simulink model "Basic_Control_Pendulum_RBF"  (R2023b)
settings: Solver=FixedStepAuto  StartTime=0.0  StopTime=20  FixedStep=0.001  RelTol=1e-3
values from neighbouring files (symbols this model uses):
  weights = weights_swarm(:,:,i)    [PSO_Optimization.m]
settings Model: Creator=Ing. Daniel Galván  LastModifiedBy=HP
settings SolverCC: AlgebraicLoopSolver=TrustRegion
settings DataIOCC: ReturnWorkspaceOutputs=off
settings DebuggingCC: UnconnectedInputMsg=warning  UnconnectedOutputMsg=warning  UnconnectedLineMsg=warning  ArithmeticOperatorsInVariantConditions=warning
settings ModelReferenceCC: EnableRefExpFcnMdlSchedulingChecks=on
settings SFSimCC: SimUseLocalCustomCode=off  CustomCodeUndefinedFunction=UseInterfaceOnly
settings RTWCC: RTWUseLocalCustomCode=off

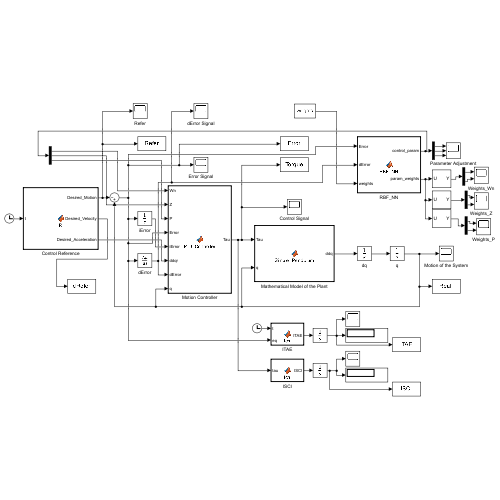
[thumbnail: Simulink's stored preview of the top-level diagram]
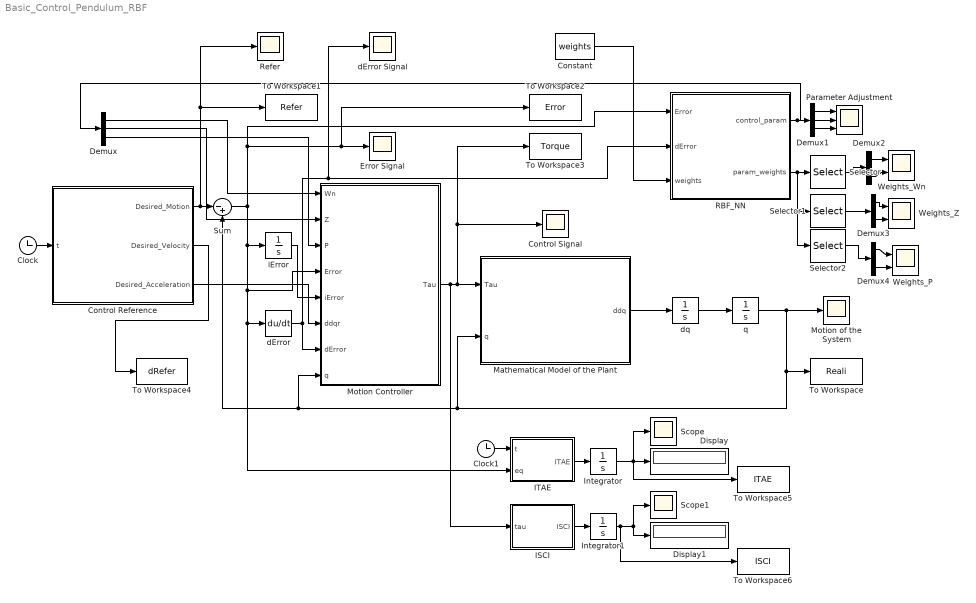
== system Basic_Control_Pendulum_RBF ==
  Clock : Clock
  Clock1 : Clock
  Constant : Constant  Value=weights
  Control Reference : MATLAB Function  TreatAsAtomicUnit=on
  Control Signal : Scope
  Demux : Demux  Outputs=3
  Demux1 : Demux  Outputs=3
  Demux2 : Demux  Outputs=2
  Demux3 : Demux  Outputs=2
  Demux4 : Demux  Outputs=2
  Display : Display
  Display1 : Display
  Error Signal : Scope
  ISCI : MATLAB Function  TreatAsAtomicUnit=on
  ITAE : MATLAB Function  TreatAsAtomicUnit=on
  Integrator : Integrator
  Integrator1 : Integrator
  Mathematical Model of the Plant : MATLAB Function  TreatAsAtomicUnit=on
  Motion Controller : MATLAB Function  TreatAsAtomicUnit=on
  Motion of the System : Scope
  Parameter Adjustment : Scope  NumInputPorts=3
  RBF_NN : MATLAB Function  TreatAsAtomicUnit=on
  Refer : Scope
  Scope : Scope
  Scope1 : Scope
  Selector : Selector  NumberOfDimensions=2  InputPortWidth=3  IndexOptions=Index vector (dialog),Index vector (dialog)  Indices=1,[1 2]  OutputSizes=1,1
  Selector1 : Selector  NumberOfDimensions=2  InputPortWidth=3  IndexOptions=Index vector (dialog),Index vector (dialog)  Indices=2,[1 2]  OutputSizes=1,1
  Selector2 : Selector  NumberOfDimensions=2  InputPortWidth=3  IndexOptions=Index vector (dialog),Index vector (dialog)  Indices=3,[1 2]  OutputSizes=1,1
  Sum : Sum  Inputs=|-+
  To Workspace : ToWorkspace  VariableName=Reali  SampleTime=-1
  To Workspace1 : ToWorkspace  VariableName=Refer  SampleTime=-1
  To Workspace2 : ToWorkspace  VariableName=Error  SampleTime=-1
  To Workspace3 : ToWorkspace  VariableName=Torque  SampleTime=-1
  To Workspace4 : ToWorkspace  VariableName=dRefer  SampleTime=-1
  To Workspace5 : ToWorkspace  VariableName=ITAE  SampleTime=-1
      settings: MaxDataPoints=1
  To Workspace6 : ToWorkspace  VariableName=ISCI  SampleTime=-1
      settings: MaxDataPoints=1
  Weights_P : Scope  NumInputPorts=2
  Weights_Wn : Scope  NumInputPorts=2
  Weights_Z : Scope  NumInputPorts=2
  dError : Derivative
  dError Signal : Scope
  dq : Integrator
  iError : Integrator
  q : Integrator
  wires:
  Clock/1 -> Control Reference/1(t)
  Mathematical Model of the Plant/1(ddq) -> dq/1
  dq/1 -> q/1
  iError/1 -> Motion Controller/5(iError)
  dError/1 -> dError Signal/1, RBF_NN/2(dError), Motion Controller/7(dError)
  q/1 -> To Workspace/1, Mathematical Model of the Plant/2(q), Sum/2, Motion Controller/8(q), Motion of the System/1
  Control Reference/1(Desired_Motion) -> Refer/1, To Workspace1/1, Sum/1
  Control Reference/3(Desired_Acceleration) -> Motion Controller/6(ddqr)
  RBF_NN/1(control_param) -> Demux/1, Demux1/1
  Demux/3 -> Motion Controller/3(P)
  Demux/2 -> Motion Controller/2(Z)
  Demux/1 -> Motion Controller/1(Wn)
  Demux1/2 -> Parameter Adjustment/2
  Demux1/1 -> Parameter Adjustment/1
  Demux1/3 -> Parameter Adjustment/3
  Control Reference/2(Desired_Velocity) -> To Workspace4/1
  RBF_NN/2(param_weights) -> Selector2/1, Selector1/1, Selector/1
  Selector/1 -> Demux2/1
  Demux2/1 -> Weights_Wn/1
  Demux2/2 -> Weights_Wn/2
  Demux3/2 -> Weights_Z/2
  Demux3/1 -> Weights_Z/1
  Selector1/1 -> Demux3/1
  Demux4/1 -> Weights_P/1
  Demux4/2 -> Weights_P/2
  Selector2/1 -> Demux4/1
  ITAE/1(ITAE) -> Integrator/1
  Integrator/1 -> To Workspace5/1, Display/1, Scope/1
  Clock1/1 -> ITAE/1(t)
  Sum/1 -> ITAE/2(eq), dError/1, Motion Controller/4(Error), iError/1, RBF_NN/1(Error), To Workspace2/1, Error Signal/1
  ISCI/1(ISCI) -> Integrator1/1
  Integrator1/1 -> To Workspace6/1, Display1/1, Scope1/1
  Constant/1 -> RBF_NN/3(weights)
  Motion Controller/1(Tau) -> ISCI/1(tau), To Workspace3/1, Control Signal/1, Mathematical Model of the Plant/1(Tau)

== matlab function Basic_Control_Pendulum_RBF/Control Reference ==
  data: Desired_Motion output size=1; t input size=1; Desired_Velocity output size=1; Desired_Acceleration output size=1
 function [Desired_Motion, Desired_Velocity, Desired_Acceleration] = R(t)

if t < 6
    [P1d, V1d, A1d] = Bezier_Reference_Profile(t, 0, 3, 0, 0.785398);
elseif t < 12
    [P1d, V1d, A1d] = Bezier_Reference_Profile(t, 6, 9, 0.785398, -0.523599);
else
    [P1d, V1d, A1d] = Bezier_Reference_Profile(t, 12, 15, -0.523599, 0);
end

Desired_Motion = P1d;

Desired_Velocity = V1d;

Desired_Acceleration = A1d;

 end

== matlab function Basic_Control_Pendulum_RBF/Mathematical Model of the Plant ==
  data: Tau input; q input; ddq output
function ddq = Simple_Pendulum(Tau, q)

m = 3.88;  lc = 0.081;
I = 0.16;   g = 9.81;

ddq = (Tau - m*g*lc*sin(q))/(m*lc^2 + I);

end

== matlab function Basic_Control_Pendulum_RBF/RBF_NN ==
  data: Error input size=1; dError input size=1; weights input; control_param output size=[3,1]; param_weights output size=[3,2,1]
function [control_param,param_weights]  = RBF_NN(Error, dError, weights)

    % Dimensions of data %%%%%%%%%%%%%%%%%%%%%%%%%%%%%%%%%%%%%%%%%%%%%%%%%%

    % number of inputs = 2
    % dim of inputs = 1
    % number of rbfs = 2
    % number of outputs = 3 x dim_inputs

    inputs = [Error,dError]; % dim_inputs x num_inputs
    
    num_inputs = 2; % = size(inputs,2);
    dim_inputs = 1; % = size(inputs,1);
    num_rbfs = 2; % = size(weights,2);
    num_outputs = 3; % = size(weights,1);


    % RBF Nets Params %%%%%%%%%%%%%%%%%%%%%%%%%%%%%%%%%%%%%%%%%%%%%%%%%%%%%

    centers = [-1, 1]; % dim_inputs x num_rbfs 

    % centers = [-1, 1; 
    %            1, -1]; % (dim_inputs x num_inputs) x num_rbfs 

    width = 2; % same for all rbfs

    % weights = [0.5, 0.2; 
    %            0.3, 0.2; 
    %            0.3, 0.1]; % num_outputs x num_rbfs

    %delta = [1e-3,1e-3,1e-3]; % 1 x num_outputs % could be same for all rbfs
    delta = [1e-3,1e-3,1e-3]; % 1 x num_outputs % could be same for all rbfs


    % RBF Online Training: Gradient Descent (Saad) %%%%%%%%%%%%%%%%%%%%%%%%

    param_Adjustments = zeros(num_outputs,dim_inputs); % num_outputs x dim_inputs
    param_weights = zeros(num_outputs,num_rbfs,dim_inputs); % num_outputs x num_rbfs x dim_inputs
    rbfOutputs = zeros(num_inputs,num_rbfs); % num_inputs x num_rbfs
    
    for j = 1:num_inputs
        rbfOutputs(j,:) = exp(-sum((inputs(:,j) - centers).^2,1) ./ (2 * width.^2)); % 1 x num_rbfs
    end

    norm_rbfOutputs = sum(rbfOutputs.^2,'all'); % 1 x 1

    % % Value by value updating
    % for ii = 1:dim_inputs % dim_inputs
    %     param_weights(:,:,ii) = weights;
    %     for i = 1:num_outputs % num_outputs
    %         for j = 1:num_inputs % num_inputs
    %             for k = 1:num_rbfs % num_rbfs
    %                 if norm_rbfOutputs ~= 0
    %                     % inputs(ii,j).*rbfOutputs(1,k); 1 x 1
    %                     param_weights(i,k,ii) = param_weights(i,k,ii) + delta(i) * inputs(ii,j)*rbfOutputs(j,k) / norm_rbfOutputs; % 1 x 1
    %                 end
    %             end
    %         end
    %     end
    %     param_Adjustments(:,ii) = sum(param_weights(:,:,ii) * rbfOutputs',2);
    % end
    
    % % Matrix form, update for num_rbfs
    % for ii = 1:dim_inputs % dim_inputs
    %     param_weights(:,:,ii) = weights;
    %     for i = 1:num_outputs % num_outputs
    %         for j = 1:num_inputs % num_inputs
    %             if norm_rbfOutputs ~= 0
    %                 % inputs(ii,j).*rbfOutputs; 1 x num_rbfs
    %                 param_weights(i,:,ii) = param_weights(i,:,ii) + delta(i).*inputs(ii,j).*rbfOutputs(j,:)./norm_rbfOutputs; %  1 x num_rbfs
    %             end
    %         end
    %     end
    %     param_Adjustments(:,ii) = sum(param_weights(:,:,ii) * rbfOutputs',2);
    % end

    % % Matrix form, update for num_rbfs, num_inputs
    % for ii = 1:dim_inputs % dim_inputs
    %     param_weights(:,:,ii) = weights;
    %     for i = 1:num_outputs % num_outputs
    %         if norm_rbfOutputs ~= 0
    %             % inputs(ii,:)'*rbfOutputs; num_inputs x num_rbfs
    %             % sum(inputs(ii,:)'*rbfOutputs,1); 1 x num_rbfs
    %             param_weights(i,:,ii) = param_weights(i,:,ii) + delta(i) .* inputs(ii,:)*rbfOutputs ./ norm_rbfOutputs; % 1 x num_rbfs
    %         end
    %     end
    %     param_Adjustments(:,ii) = sum(param_weights(:,:,ii) * rbfOutputs',2);
    % end

    % Matrix form, update for num_rbfs, num_inputs, num_outputs
    for ii = 1:dim_inputs % dim_inputs
        param_weights(:,:,ii) = weights;
        if norm_rbfOutputs ~= 0
            % inputs(ii,:)*rbfOutputs; num_inputs x num_rbfs
            % sum(inputs(ii,:)*rbfOutputs,1); 1 x num_rbfs
            param_weights(:,:,ii) = param_weights(:,:,ii) + delta' * inputs(ii,:)*rbfOutputs ./ norm_rbfOutputs; % 1 x num_rbfs
        end
        param_Adjustments(:,ii) = sum(param_weights(:,:,ii) * rbfOutputs',2);
    end

    control_param = param_Adjustments;

end

== matlab function Basic_Control_Pendulum_RBF/Motion Controller ==
  data: Wn input; Z input; P input; Error input; iError input; ddqr input; dError input; q input; Tau output
function Tau  = PID_Controller(Wn, Z, P, Error, iError, ddqr, dError, q)

m = 3.88;  lc = 0.081;
I = 0.16;   g = 9.81;

% Wn = 3;
%  Z = 0.707;  
%  P = 0.1;

kp = Wn^2 + 2*P*Z*Wn;  kd = P + 2*Z*Wn;  
ki = P*Wn;

Tau = (m*lc^2 + I)*(ddqr - kp*Error - kd*dError - ki*iError)  + (m*g*lc)*sin(q);

end

== matlab function Basic_Control_Pendulum_RBF/ITAE ==
  data: t input; ITAE output; eq input
function ITAE = fcn(t,eq)

ITAE = t.*abs(eq);

== matlab function Basic_Control_Pendulum_RBF/ISCI ==
  data: tau input; ISCI output
function ISCI = fcn(tau)

ISCI = tau.^2;
